simulink model "electricVehicle_closedLoop"  (R2015a)
settings: Solver=ode23t  StartTime=0.0  StopTime=100  RelTol=1e-3  AbsTol=1e-3
PreLoadFcn:
  | car_tire_data
  | load engine_data
undefined symbols (not defined in the file or in its folder): rider_mass, sigbuilder_block, tire_dia, vehicle_mass
libraries: fl_lib x118, nesl_utility x16, sdl_lib x11, simulink x4, elec_lib x1
(part 1 of 2)
settings Model: Creator=sseshadr  LastModifiedBy=chahn
settings SimscapeCC: SimscapeLogType=all  SimscapeLogDataHistory=10000

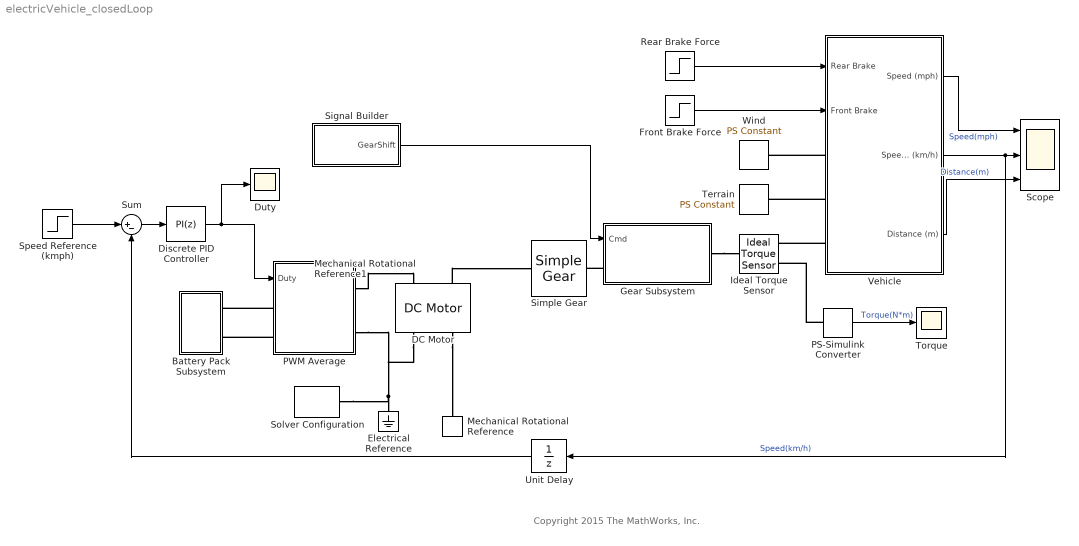
== system electricVehicle_closedLoop ==
  note: Copyright 2015 The MathWorks, Inc.
  Battery Pack Subsystem : Subsystem
  DC Motor : elec_lib/Actuators & Drivers/Rotational Actuators/DC Motor  parameterization=1  Ra=0.0093 Ohm  La=172 uH  emf_or_torque=2  Kv=0.19 V/(rad/s)  Ki=0.19 N*m/A  T_stall=2.4e-4 N*m  w_max=1.91e+4 rpm  w_rated=1.5e+4 rpm  P_rated=0.08 W  V_rated=1.5 V  J=0.001 kg*m^2  lam_param=1  lam=1e-6 N*m/(rad/s)  i_noload=0 A  V_i_noload=1.5 V  speed0=0 rad/s  alpha=0.00393 1/K  Tmeas=25 C  thermal_mass=100 J/K  initial_temperature=25 C
  Discrete PID Controller : simulink/Continuous/PID Controller  Controller=PI  TimeDomain=Discrete-time  SampleTime=0.05  IntegratorMethod=Forward Euler  FilterMethod=Forward Euler  Form=Parallel  UseFilter=on  ControllerParametersSource=internal  P=0.1  I=0.05  D=0  N=100  InitialConditionSource=internal  InitialConditionForIntegrator=0  InitialConditionForFilter=0  ExternalReset=none  LimitOutput=on  UpperSaturationLimit=1  LowerSaturationLimit=0  LinearizeAsGain=off  AntiWindupMode=none  Kb=1  TrackingMode=off  Kt=1  PParamMin=[]  PParamMax=[]  IParamMin=[]  IParamMax=[]  DParamMin=[]  DParamMax=[]  NParamMin=[]  NParamMax=[]  KbParamMin=[]  KbParamMax=[]  KtParamMin=[]  KtParamMax=[]  POutMin=[]  POutMax=[]  IOutMin=[]  IOutMax=[]  DOutMin=[]  DOutMax=[]  NOutMin=[]  NOutMax=[]  KbOutMin=[]  KbOutMax=[]  KtOutMin=[]  KtOutMax=[]  IntegratorOutMin=[]  IntegratorOutMax=[]  FilterOutMin=[]  FilterOutMax=[]  SumOutMin=[]  SumOutMax=[]  SumI1OutMin=[]  SumI1OutMax=[]  SumI2OutMin=[]  SumI2OutMax=[]  SumI3OutMin=[]  SumI3OutMax=[]  SumDOutMin=[]  SumDOutMax=[]  SaturationOutMin=[]  SaturationOutMax=[]  IntegratorContinuousStateAttributes=''  IntegratorStateMustResolveToSignalObject=off  IntegratorRTWStateStorageClass=Auto  FilterContinuousStateAttributes=''  FilterStateMustResolveToSignalObject=off  FilterRTWStateStorageClass=Auto  DifferentiatorICPrevScaledInput=0  DifferentiatorOutMin=[]  DifferentiatorOutMax=[]
  Duty : Scope
      settings: TimeRange=40  LimitDataPoints=on  MaxDataPoints=5000  SaveToWorkspace=off  SaveName=ScopeData4  YMin=0  YMax=1000  SampleTime=-1
  Electrical Reference : fl_lib/Electrical/Electrical Elements/Electrical Reference
  Front Brake Force : Step  Time=75  After=1000  SampleTime=0
      settings: AttributesFormatString=%<After> N at %<Time> s
  Gear Subsystem : Subsystem
  Ideal Torque Sensor : fl_lib/Mechanical/Mechanical Sensors/Ideal Torque Sensor
  Mechanical Rotational Reference : fl_lib/Mechanical/Rotational Elements/Mechanical Rotational Reference
  Mechanical Rotational Reference1 : fl_lib/Mechanical/Rotational Elements/Mechanical Rotational Reference
  PS-Simulink Converter : nesl_utility/PS-Simulink Converter  PhysicalDomain=network_engine_domain  SubClassName=ps_output  LeftPortType=input  RightPortType=output  PseudoPeriodic=off  Frequencies=[]  Unit=N*m  AffineConversion=off
  PWM Average : Subsystem
  Rear Brake Force : Step  Time=50  After=500  SampleTime=0
      settings: AttributesFormatString=%<After> N at %<Time> s
  Scope : Scope  NumInputPorts=3
      settings: TimeRange=auto  MaxDataPoints=5000  SaveToWorkspace=off  YMin=-5~-5~-5  YMax=5~5~5  SampleTime=-1  DataFormat=Array
  Signal Builder : Subsystem  Tag=STV Subsys  LoadFcn=sigbuilder_block('load');  StartFcn=sigbuilder_block('start');  StopFcn=sigbuilder_block('stop');  ClipboardFcn=sigbuilder_block('clipboard');  mask(Sigbuilder block){}
      mask help: Simulink:masks:SigbuilderBlock_MD
      mask init:
      | if ~strcmp(get_param(bdroot(gcbh),'SimulationStatus'),'stopped') tuvar = sigbuilder_block('maskInit'); end
      settings: CopyFcn=sigbuilder_block('copy');  DeleteFcn=sigbuilder_block('delete');  ModelCloseFcn=sigbuilder_block('modelClose');  PreSaveFcn=sigbuilder_block('preSave');  PauseFcn=sigbuilder_block('pause');  ContinueFcn=sigbuilder_block('continue');  NameChangeFcn=sigbuilder_block('namechange');  OpenFcn=sigbuilder_block('open',[306 225.75 549.75 399.75 ]);  CloseFcn=sigbuilder_block('close');
      mask Display: plot(0, 0, 100, 100,[2, 2, 32, 32, 2], [68, 8, 8, 68, 68],[32, 2], [38, 38], [32, 19, 2],[53, 60, 44], [32, 17, 17, 2],[16, 16, 31, 31]);txt = getActiveGroup(gcbh);text(2, 100, txt,'verticalAlignment', 'top');
  Simple Gear : sdl_lib/Gears/Simple Gear  ratio=12  rotation_direction=1  friction_model=1  T_noload=0.1 N*m  T_nom=5 N*m  efficiency_nom=0.8  efficiency=0.8  mu_visc=[ 0 0 ] N*m/(rad/s)  w_thr=0.01 rad/s  temperature_TLU=[ 280 300 320 ] K  load_TLU=[ 1 5 10 ] N*m  efficiency_TLU=[ 0.95 0.9 0.85 ]  efficiency_TLU2=[ 0.85 0.8 0.75; 0.95 0.9 0.85; 0.85 0.8 0.7 ]  thermal_mass=50 J/K  T_init=300 K
  Solver Configuration : nesl_utility/Solver Configuration  PhysicalDomain=network_engine_domain  SubClassName=solver  LeftPortType=input  RightPortType=generic  Accelerate=off  Tones=[]  Harmonics=[]  SimulateNoise=off  Profile=off  UseLocalSampling=off  EnableSwitchedLinearOptims=on  FrequencyDomain=off  UseCCode=off  RelTol=0.001  AbsTol=1e-06  MinStep=1e-09  ToWorkspace=off  RevertToSquareIcSolve=off  NumHomotopyIterations=100  PhasorMode=off  PhasorModeNumHarmonics=1  DoDC=off  ResidualTolerance=1e-09  UseLocalSolver=off  LocalSolverChoice=NE_BACKWARD_EULER_ADVANCER  LocalSolverSampleTime=1e-7  DoFixedCost=off  MaxNonlinIter=3  MaxModeIter=2  LinearAlgebra=Sparse  DelaysMemoryBudget=1024  AutomaticFiltering=on  FilteringTimeConstant=0.001
  Speed Reference (kmph) : Step  Time=30  Before=40  After=5  SampleTime=0
      settings: AttributesFormatString=%<Before> to %<After> at %<Time>s
  Sum : Sum  Inputs=|+-
  Terrain : fl_lib/Physical Signals/Sources/PS Constant  constant=0
  Torque : Scope
      settings: TimeRange=40  LimitDataPoints=on  MaxDataPoints=5000  SaveToWorkspace=off  SaveName=ScopeData2  YMin=0  YMax=1000  SampleTime=-1
  Unit Delay : UnitDelay  SampleTime=0.05
  Vehicle : Subsystem
  Wind : fl_lib/Physical Signals/Sources/PS Constant  constant=0
  wires:
  Rear Brake Force/1 -> Vehicle/1(Rear Brake)
  Vehicle/1(Speed (mph)) -> Scope/1  "Speed(mph)"
  Vehicle/2(Speed (km/h)) -> Unit Delay/1, Scope/2  "Speed(km/h)"
  Vehicle/3(Distance (m)) -> Scope/3  "Distance(m)"
  Front Brake Force/1 -> Vehicle/2(Front Brake)
  PS-Simulink Converter/1 -> Torque/1  "Torque(N*m)"
  Signal Builder/1(GearShift) -> Gear Subsystem/1(Cmd)
  Speed Reference (kmph)/1 -> Sum/1
  Sum/1 -> Discrete PID Controller/1
  Discrete PID Controller/1 -> Duty/1, PWM Average/1(Duty)
  Unit Delay/1 -> Sum/2
  connections:
  Vehicle/LConn1 -- Wind/RConn1
  Vehicle/LConn2 -- Terrain/RConn1
  Vehicle/LConn3 -- Ideal Torque Sensor/RConn1
  PS-Simulink Converter/LConn1 -- Ideal Torque Sensor/RConn2
  Gear Subsystem/RConn1 -- Ideal Torque Sensor/LConn1
  DC Motor/LConn2 -- Simple Gear/LConn1
  Gear Subsystem/LConn1 -- Simple Gear/RConn1
  DC Motor/RConn2 -- Mechanical Rotational Reference/LConn1
  Electrical Reference/LConn1 -- Solver Configuration/RConn1 -- DC Motor/RConn1 -- PWM Average/RConn2
  PWM Average/RConn1 -- DC Motor/LConn1
  PWM Average/LConn1 -- Battery Pack Subsystem/RConn1
  PWM Average/LConn2 -- Battery Pack Subsystem/RConn2

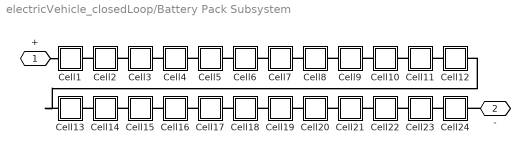
== system electricVehicle_closedLoop/Battery Pack Subsystem ==
  Cell1 : Subsystem
  Cell10 : Subsystem
  Cell11 : Subsystem
  Cell12 : Subsystem
  Cell13 : Subsystem
  Cell14 : Subsystem
  Cell15 : Subsystem
  Cell16 : Subsystem
  Cell17 : Subsystem
  Cell18 : Subsystem
  Cell19 : Subsystem
  Cell2 : Subsystem
  Cell20 : Subsystem
  Cell21 : Subsystem
  Cell22 : Subsystem
  Cell23 : Subsystem
  Cell24 : Subsystem
  Cell3 : Subsystem
  Cell4 : Subsystem
  Cell5 : Subsystem
  Cell6 : Subsystem
  Cell7 : Subsystem
  Cell8 : Subsystem
  Cell9 : Subsystem
  + : PMIOPort  Port=1  Side=Right
  - : PMIOPort  Port=2  Side=Right
  connections:
  +/RConn1 -- Cell1/LConn1
  Cell2/LConn1 -- Cell1/RConn1
  -/RConn1 -- Cell24/RConn1
  Cell3/LConn1 -- Cell2/RConn1
  Cell4/LConn1 -- Cell3/RConn1
  Cell5/LConn1 -- Cell4/RConn1
  Cell6/LConn1 -- Cell5/RConn1
  Cell7/LConn1 -- Cell6/RConn1
  Cell8/LConn1 -- Cell7/RConn1
  Cell9/LConn1 -- Cell8/RConn1
  Cell10/LConn1 -- Cell9/RConn1
  Cell11/LConn1 -- Cell10/RConn1
  Cell12/LConn1 -- Cell11/RConn1
  Cell18/LConn1 -- Cell17/RConn1
  Cell20/LConn1 -- Cell19/RConn1
  Cell15/LConn1 -- Cell14/RConn1
  Cell22/LConn1 -- Cell21/RConn1
  Cell24/LConn1 -- Cell23/RConn1
  Cell23/LConn1 -- Cell22/RConn1
  Cell19/LConn1 -- Cell18/RConn1
  Cell14/LConn1 -- Cell13/RConn1
  Cell21/LConn1 -- Cell20/RConn1
  Cell17/LConn1 -- Cell16/RConn1
  Cell16/LConn1 -- Cell15/RConn1
  Cell13/LConn1 -- Cell12/RConn1

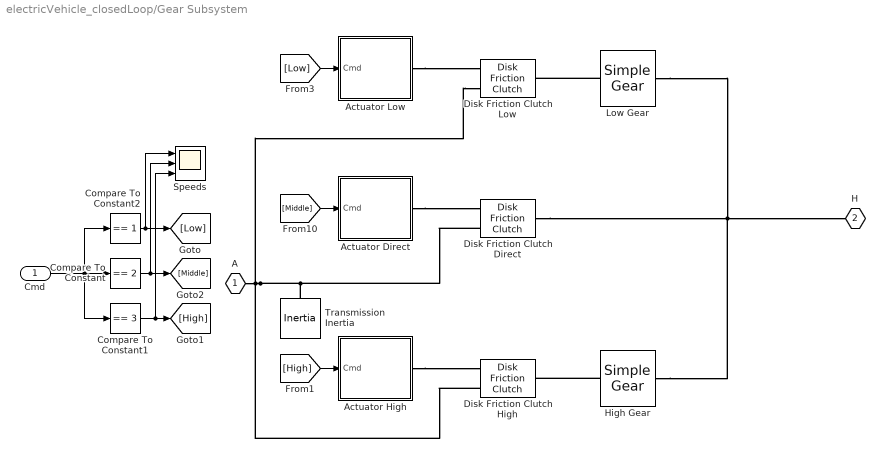
== system electricVehicle_closedLoop/Gear Subsystem ==
  Cmd : Inport
  Actuator Direct : Subsystem
  Actuator High : Subsystem
  Actuator Low : Subsystem
  Compare To Constant : simulink/Logic and Bit Operations/Compare To Constant  relop===  const=2  OutDataTypeStr=boolean
  Compare To Constant1 : simulink/Logic and Bit Operations/Compare To Constant  relop===  const=3  OutDataTypeStr=boolean
  Compare To Constant2 : simulink/Logic and Bit Operations/Compare To Constant  relop===  const=1  OutDataTypeStr=boolean
  Disk Friction Clutch Direct : sdl_lib/Clutches/Disk Friction Clutch  geometry_model=1  r_eff=130 mm  d_o=150 mm  d_i=100 mm  nS=4  piston_area=0.001 m^2  unidirectional=0  friction_model=1  mu_coulomb=0.3  mu_w_vector=[ 0 0.1 0.2 0.3 0.4 0.5 1 2 5 10 100 1000 ] rad/s  mu_coulomb_vector=[ 0.29 0.28 0.26 0.22 0.21 0.2 0.2 0.19 0.19 0.19 0.19 0.19 ]  mu_interp_method=1  mu_extrap_method=1  mu_static=0.35  d_f=1  w_tol=0.001 rad/s  pressure_min=100 Pa  mu_visc=0 N*m/(rad/s)  initial_state_locked=0
  Disk Friction Clutch High : sdl_lib/Clutches/Disk Friction Clutch  geometry_model=1  r_eff=130 mm  d_o=150 mm  d_i=100 mm  nS=4  piston_area=0.001 m^2  unidirectional=0  friction_model=1  mu_coulomb=0.3  mu_w_vector=[ 0 0.1 0.2 0.3 0.4 0.5 1 2 5 10 100 1000 ] rad/s  mu_coulomb_vector=[ 0.29 0.28 0.26 0.22 0.21 0.2 0.2 0.19 0.19 0.19 0.19 0.19 ]  mu_interp_method=1  mu_extrap_method=1  mu_static=0.35  d_f=1  w_tol=0.001 rad/s  pressure_min=100 Pa  mu_visc=0 N*m/(rad/s)  initial_state_locked=0
  Disk Friction Clutch Low : sdl_lib/Clutches/Disk Friction Clutch  geometry_model=1  r_eff=130 mm  d_o=150 mm  d_i=100 mm  nS=4  piston_area=0.001 m^2  unidirectional=0  friction_model=1  mu_coulomb=0.3  mu_w_vector=[ 0 0.1 0.2 0.3 0.4 0.5 1 2 5 10 100 1000 ] rad/s  mu_coulomb_vector=[ 0.29 0.28 0.26 0.22 0.21 0.2 0.2 0.19 0.19 0.19 0.19 0.19 ]  mu_interp_method=1  mu_extrap_method=1  mu_static=0.35  d_f=1  w_tol=0.001 rad/s  pressure_min=100 Pa  mu_visc=0 N*m/(rad/s)  initial_state_locked=0
  High Gear : sdl_lib/Gears/Simple Gear  ratio=0.67  rotation_direction=1  friction_model=1  T_noload=0.1 N*m  T_nom=5 N*m  efficiency_nom=0.8  efficiency=0.8  mu_visc=[ 0 0 ] N*m/(rad/s)  w_thr=0.01 rad/s  temperature_TLU=[ 280 300 320 ] K  load_TLU=[ 1 5 10 ] N*m  efficiency_TLU=[ 0.95 0.9 0.85 ]  efficiency_TLU2=[ 0.85 0.8 0.75; 0.95 0.9 0.85; 0.85 0.8 0.7 ]  thermal_mass=50 J/K  T_init=300 K
  Low Gear : sdl_lib/Gears/Simple Gear  ratio=1.5  rotation_direction=1  friction_model=1  T_noload=0.1 N*m  T_nom=5 N*m  efficiency_nom=0.8  efficiency=0.8  mu_visc=[ 0 0 ] N*m/(rad/s)  w_thr=0.01 rad/s  temperature_TLU=[ 280 300 320 ] K  load_TLU=[ 1 5 10 ] N*m  efficiency_TLU=[ 0.95 0.9 0.85 ]  efficiency_TLU2=[ 0.85 0.8 0.75; 0.95 0.9 0.85; 0.85 0.8 0.7 ]  thermal_mass=50 J/K  T_init=300 K
  Speeds : Scope  NumInputPorts=3
      settings: TimeRange=auto  MaxDataPoints=5000  SaveToWorkspace=off  YMin=-0.2~0~-5  YMax=1.7~2~5  SampleTime=-1
  Transmission Inertia : fl_lib/Mechanical/Rotational Elements/Inertia  inertia=0.0005 kg*m^2  w_specify=off  w_priority=High  w=0 rad/s  t_specify=off  t_priority=High  t=0 N*m
  A : PMIOPort  Port=1  Side=Left
  H : PMIOPort  Port=2  Side=Right
  wires:
  [High] -> Actuator High/1(Cmd)
  [Low] -> Actuator Low/1(Cmd)
  [Middle] -> Actuator Direct/1(Cmd)
  Cmd/1 -> Compare To Constant1/1, Compare To Constant2/1, Compare To Constant/1
  Compare To Constant2/1 -> Speeds/1, [Low]
  Compare To Constant/1 -> Speeds/2, [Middle]
  Compare To Constant1/1 -> Speeds/3, [High]
  connections:
  High Gear/LConn1 -- Disk Friction Clutch High/RConn1
  Actuator High/RConn1 -- Disk Friction Clutch High/LConn1
  Disk Friction Clutch Low/LConn2 -- Disk Friction Clutch High/LConn2 -- Transmission Inertia/LConn1 -- Disk Friction Clutch Direct/LConn2 -- A/RConn1
  Actuator Low/RConn1 -- Disk Friction Clutch Low/LConn1
  Low Gear/LConn1 -- Disk Friction Clutch Low/RConn1
  Actuator Direct/RConn1 -- Disk Friction Clutch Direct/LConn1
  Disk Friction Clutch Direct/RConn1 -- Low Gear/RConn1 -- H/RConn1 -- High Gear/RConn1

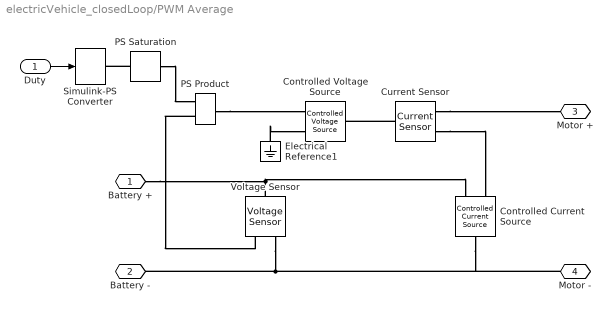
== system electricVehicle_closedLoop/PWM Average ==
  Duty : Inport
  Controlled Current Source : fl_lib/Electrical/Electrical Sources/Controlled Current Source
  Controlled Voltage Source : fl_lib/Electrical/Electrical Sources/Controlled Voltage Source
  Current Sensor : fl_lib/Electrical/Electrical Sensors/Current Sensor
  Electrical Reference1 : fl_lib/Electrical/Electrical Elements/Electrical Reference
  PS Product : fl_lib/Physical Signals/Functions/PS Product
  PS Saturation : fl_lib/Physical Signals/Nonlinear Operators/PS Saturation  upper_limit=1  lower_limit=0
  Simulink-PS Converter : nesl_utility/Simulink-PS Converter  PhysicalDomain=network_engine_domain  SubClassName=ps_input  LeftPortType=input  RightPortType=output  PseudoPeriodic=off  Frequencies=[]  NoiseDistribution=none  NoiseParameters=[]  Unit=1  AffineConversion=off  InputFiltering=off  SimscapeFilterOrder=1  InputFilterTimeConstant=0.001  UdotUserProvided=1
  Voltage Sensor : fl_lib/Electrical/Electrical Sensors/Voltage Sensor
  Battery + : PMIOPort  Port=1  Side=Left
  Battery - : PMIOPort  Port=2  Side=Left
  Motor + : PMIOPort  Port=3  Side=Right
  Motor - : PMIOPort  Port=4  Side=Right
  wires:
  Duty/1 -> Simulink-PS Converter/1
  connections:
  Electrical Reference1/LConn1 -- Controlled Voltage Source/RConn2
  Current Sensor/LConn1 -- Controlled Voltage Source/LConn1
  Voltage Sensor/RConn2 -- Controlled Current Source/LConn1 -- Motor -/RConn1 -- Battery -/RConn1
  Current Sensor/RConn1 -- Controlled Current Source/RConn1
  PS Product/LConn2 -- Voltage Sensor/RConn1
  Voltage Sensor/LConn1 -- Battery +/RConn1 -- Controlled Current Source/RConn2
  PS Product/RConn1 -- Controlled Voltage Source/RConn1
  Current Sensor/RConn2 -- Motor +/RConn1
  PS Saturation/RConn1 -- PS Product/LConn1
  PS Saturation/LConn1 -- Simulink-PS Converter/RConn1

== system electricVehicle_closedLoop/Signal Builder ==
  Demux : Demux  Tag=STV Demux  Outputs=1
  FromWs : FromWorkspace  Tag=STV FromWs  VariableName=tuvar  SampleTime=0
      SigBuilderData=|
      | common.afterFinalStr = 'Extrapolate'
      | common.sampleTime = 0
      | dataSet.timeRange = [0 30]
      | dataSet.name = 'Gear'
      | sbobj.Groups.Name = 'Gear'
      | sbobj.Groups.Signals.Name = 'GearShift'
      | sbobj.Groups.Signals.XData = [0 10 10 20 20 30]
      | sbobj.Groups.Signals.YData = [1 1 2 2 3 3]
      | sbobj.Groups.TimeRange = [0 30]
  GearShift : Outport  Tag=STV Outport
  wires:
  FromWs/1 -> Demux/1
  Demux/1 -> GearShift/1

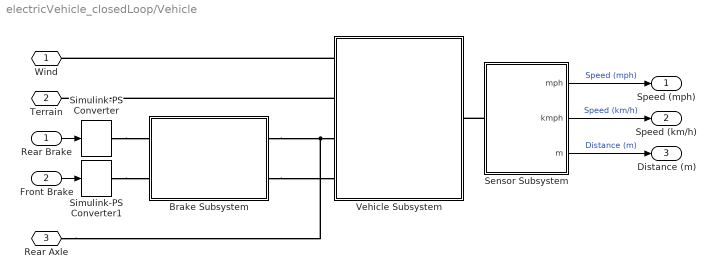
== system electricVehicle_closedLoop/Vehicle ==
  Rear Brake : Inport
  Front Brake : Inport  Port=2
  Brake Subsystem : Subsystem
  Sensor Subsystem : Subsystem
  Simulink-PS Converter : nesl_utility/Simulink-PS Converter  PhysicalDomain=network_engine_domain  SubClassName=ps_input  LeftPortType=input  RightPortType=output  PseudoPeriodic=off  Frequencies=[]  NoiseDistribution=none  NoiseParameters=[]  Unit=1  AffineConversion=off  InputFiltering=on  SimscapeFilterOrder=1  InputFilterTimeConstant=0.001  UdotUserProvided=1
  Simulink-PS Converter1 : nesl_utility/Simulink-PS Converter  PhysicalDomain=network_engine_domain  SubClassName=ps_input  LeftPortType=input  RightPortType=output  PseudoPeriodic=off  Frequencies=[]  NoiseDistribution=none  NoiseParameters=[]  Unit=1  AffineConversion=off  InputFiltering=on  SimscapeFilterOrder=1  InputFilterTimeConstant=0.001  UdotUserProvided=1
  Vehicle Subsystem : Subsystem
  Wind : PMIOPort  Port=1  Side=Left
  Terrain : PMIOPort  Port=2  Side=Left
  Rear Axle : PMIOPort  Port=3  Side=Left
  Speed (mph) : Outport
  Speed (km/h) : Outport  Port=2
  Distance (m) : Outport  Port=3
  wires:
  Sensor Subsystem/1(mph) -> Speed (mph)/1  "Speed (mph)"
  Sensor Subsystem/2(kmph) -> Speed (km/h)/1  "Speed (km/h)"
  Sensor Subsystem/3(m) -> Distance (m)/1  "Distance (m)"
  Rear Brake/1 -> Simulink-PS Converter/1
  Front Brake/1 -> Simulink-PS Converter1/1
  connections:
  Simulink-PS Converter/RConn1 -- Brake Subsystem/LConn1
  Brake Subsystem/RConn1 -- Rear Axle/RConn1 -- Vehicle Subsystem/LConn3
  Brake Subsystem/RConn2 -- Vehicle Subsystem/LConn4
  Simulink-PS Converter1/RConn1 -- Brake Subsystem/LConn2
  Sensor Subsystem/LConn1 -- Vehicle Subsystem/RConn1
  Vehicle Subsystem/LConn1 -- Wind/RConn1
  Vehicle Subsystem/LConn2 -- Terrain/RConn1

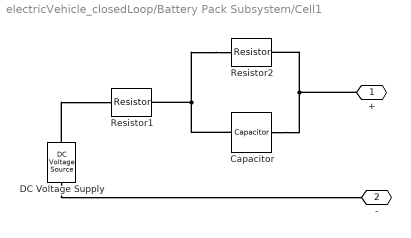
== system electricVehicle_closedLoop/Battery Pack Subsystem/Cell1 ==
  Capacitor : fl_lib/Electrical/Electrical Elements/Capacitor  c=5000 F  r=1e-6 Ohm  g=0 1/Ohm  i_specify=off  i_priority=High  i=0 A  v_specify=off  v_priority=High  v=0 V  vc_specify=on  vc_priority=High  vc=0 V
  DC Voltage Supply : fl_lib/Electrical/Electrical Sources/DC Voltage Source  v0=4.2 V
  Resistor1 : fl_lib/Electrical/Electrical Elements/Resistor  R=0.01 Ohm  i_specify=off  i_priority=High  i=0 A  v_specify=off  v_priority=High  v=0 V
  Resistor2 : fl_lib/Electrical/Electrical Elements/Resistor  R=0.005 Ohm  i_specify=off  i_priority=High  i=0 A  v_specify=off  v_priority=High  v=0 V
  + : PMIOPort  Port=1  Side=Left
  - : PMIOPort  Port=2  Side=Right
  connections:
  Resistor2/LConn1 -- Capacitor/LConn1 -- Resistor1/RConn1
  DC Voltage Supply/RConn1 -- -/RConn1
  Resistor2/RConn1 -- +/RConn1 -- Capacitor/RConn1
  DC Voltage Supply/LConn1 -- Resistor1/LConn1

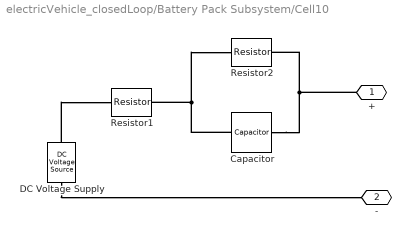
== system electricVehicle_closedLoop/Battery Pack Subsystem/Cell10 ==
  Capacitor : fl_lib/Electrical/Electrical Elements/Capacitor  c=5000 F  r=1e-6 Ohm  g=0 1/Ohm  i_specify=off  i_priority=High  i=0 A  v_specify=off  v_priority=High  v=0 V  vc_specify=on  vc_priority=High  vc=0 V
  DC Voltage Supply : fl_lib/Electrical/Electrical Sources/DC Voltage Source  v0=4.2 V
  Resistor1 : fl_lib/Electrical/Electrical Elements/Resistor  R=0.01 Ohm  i_specify=off  i_priority=High  i=0 A  v_specify=off  v_priority=High  v=0 V
  Resistor2 : fl_lib/Electrical/Electrical Elements/Resistor  R=0.005 Ohm  i_specify=off  i_priority=High  i=0 A  v_specify=off  v_priority=High  v=0 V
  + : PMIOPort  Port=1  Side=Left
  - : PMIOPort  Port=2  Side=Right
  connections:
  DC Voltage Supply/LConn1 -- Resistor1/LConn1
  Capacitor/RConn1 -- +/RConn1 -- Resistor2/RConn1
  DC Voltage Supply/RConn1 -- -/RConn1
  Resistor1/RConn1 -- Capacitor/LConn1 -- Resistor2/LConn1

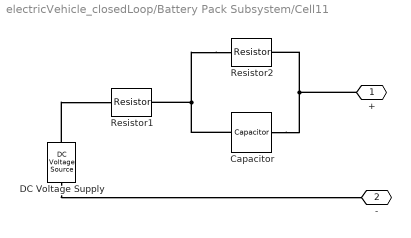
== system electricVehicle_closedLoop/Battery Pack Subsystem/Cell11 ==
  Capacitor : fl_lib/Electrical/Electrical Elements/Capacitor  c=5000 F  r=1e-6 Ohm  g=0 1/Ohm  i_specify=off  i_priority=High  i=0 A  v_specify=off  v_priority=High  v=0 V  vc_specify=on  vc_priority=High  vc=0 V
  DC Voltage Supply : fl_lib/Electrical/Electrical Sources/DC Voltage Source  v0=4.2 V
  Resistor1 : fl_lib/Electrical/Electrical Elements/Resistor  R=0.01 Ohm  i_specify=off  i_priority=High  i=0 A  v_specify=off  v_priority=High  v=0 V
  Resistor2 : fl_lib/Electrical/Electrical Elements/Resistor  R=0.005 Ohm  i_specify=off  i_priority=High  i=0 A  v_specify=off  v_priority=High  v=0 V
  + : PMIOPort  Port=1  Side=Left
  - : PMIOPort  Port=2  Side=Right
  connections:
  Resistor2/LConn1 -- Capacitor/LConn1 -- Resistor1/RConn1
  DC Voltage Supply/RConn1 -- -/RConn1
  Resistor2/RConn1 -- +/RConn1 -- Capacitor/RConn1
  DC Voltage Supply/LConn1 -- Resistor1/LConn1

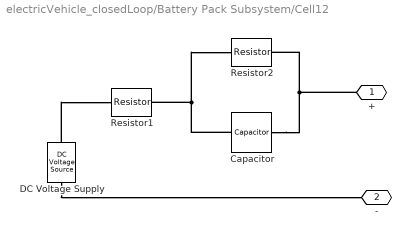
== system electricVehicle_closedLoop/Battery Pack Subsystem/Cell12 ==
  Capacitor : fl_lib/Electrical/Electrical Elements/Capacitor  c=5000 F  r=1e-6 Ohm  g=0 1/Ohm  i_specify=off  i_priority=High  i=0 A  v_specify=off  v_priority=High  v=0 V  vc_specify=on  vc_priority=High  vc=0 V
  DC Voltage Supply : fl_lib/Electrical/Electrical Sources/DC Voltage Source  v0=4.2 V
  Resistor1 : fl_lib/Electrical/Electrical Elements/Resistor  R=0.01 Ohm  i_specify=off  i_priority=High  i=0 A  v_specify=off  v_priority=High  v=0 V
  Resistor2 : fl_lib/Electrical/Electrical Elements/Resistor  R=0.005 Ohm  i_specify=off  i_priority=High  i=0 A  v_specify=off  v_priority=High  v=0 V
  + : PMIOPort  Port=1  Side=Left
  - : PMIOPort  Port=2  Side=Right
  connections:
  DC Voltage Supply/LConn1 -- Resistor1/LConn1
  Capacitor/RConn1 -- +/RConn1 -- Resistor2/RConn1
  DC Voltage Supply/RConn1 -- -/RConn1
  Resistor1/RConn1 -- Capacitor/LConn1 -- Resistor2/LConn1

== system electricVehicle_closedLoop/Battery Pack Subsystem/Cell13 ==
  Capacitor : fl_lib/Electrical/Electrical Elements/Capacitor  c=5000 F  r=1e-6 Ohm  g=0 1/Ohm  i_specify=off  i_priority=High  i=0 A  v_specify=off  v_priority=High  v=0 V  vc_specify=on  vc_priority=High  vc=0 V
  DC Voltage Supply : fl_lib/Electrical/Electrical Sources/DC Voltage Source  v0=4.2 V
  Resistor1 : fl_lib/Electrical/Electrical Elements/Resistor  R=0.01 Ohm  i_specify=off  i_priority=High  i=0 A  v_specify=off  v_priority=High  v=0 V
  Resistor2 : fl_lib/Electrical/Electrical Elements/Resistor  R=0.005 Ohm  i_specify=off  i_priority=High  i=0 A  v_specify=off  v_priority=High  v=0 V
  + : PMIOPort  Port=1  Side=Left
  - : PMIOPort  Port=2  Side=Right
  connections:
  Resistor2/LConn1 -- Capacitor/LConn1 -- Resistor1/RConn1
  DC Voltage Supply/RConn1 -- -/RConn1
  Resistor2/RConn1 -- +/RConn1 -- Capacitor/RConn1
  DC Voltage Supply/LConn1 -- Resistor1/LConn1

== system electricVehicle_closedLoop/Battery Pack Subsystem/Cell14 ==
  Capacitor : fl_lib/Electrical/Electrical Elements/Capacitor  c=5000 F  r=1e-6 Ohm  g=0 1/Ohm  i_specify=off  i_priority=High  i=0 A  v_specify=off  v_priority=High  v=0 V  vc_specify=on  vc_priority=High  vc=0 V
  DC Voltage Supply : fl_lib/Electrical/Electrical Sources/DC Voltage Source  v0=4.2 V
  Resistor1 : fl_lib/Electrical/Electrical Elements/Resistor  R=0.01 Ohm  i_specify=off  i_priority=High  i=0 A  v_specify=off  v_priority=High  v=0 V
  Resistor2 : fl_lib/Electrical/Electrical Elements/Resistor  R=0.005 Ohm  i_specify=off  i_priority=High  i=0 A  v_specify=off  v_priority=High  v=0 V
  + : PMIOPort  Port=1  Side=Left
  - : PMIOPort  Port=2  Side=Right
  connections:
  DC Voltage Supply/LConn1 -- Resistor1/LConn1
  Capacitor/RConn1 -- +/RConn1 -- Resistor2/RConn1
  DC Voltage Supply/RConn1 -- -/RConn1
  Resistor1/RConn1 -- Capacitor/LConn1 -- Resistor2/LConn1

== system electricVehicle_closedLoop/Battery Pack Subsystem/Cell15 ==
  Capacitor : fl_lib/Electrical/Electrical Elements/Capacitor  c=5000 F  r=1e-6 Ohm  g=0 1/Ohm  i_specify=off  i_priority=High  i=0 A  v_specify=off  v_priority=High  v=0 V  vc_specify=on  vc_priority=High  vc=0 V
  DC Voltage Supply : fl_lib/Electrical/Electrical Sources/DC Voltage Source  v0=4.2 V
  Resistor1 : fl_lib/Electrical/Electrical Elements/Resistor  R=0.01 Ohm  i_specify=off  i_priority=High  i=0 A  v_specify=off  v_priority=High  v=0 V
  Resistor2 : fl_lib/Electrical/Electrical Elements/Resistor  R=0.005 Ohm  i_specify=off  i_priority=High  i=0 A  v_specify=off  v_priority=High  v=0 V
  + : PMIOPort  Port=1  Side=Left
  - : PMIOPort  Port=2  Side=Right
  connections:
  Resistor2/LConn1 -- Capacitor/LConn1 -- Resistor1/RConn1
  DC Voltage Supply/RConn1 -- -/RConn1
  Resistor2/RConn1 -- +/RConn1 -- Capacitor/RConn1
  DC Voltage Supply/LConn1 -- Resistor1/LConn1

== system electricVehicle_closedLoop/Battery Pack Subsystem/Cell16 ==
  Capacitor : fl_lib/Electrical/Electrical Elements/Capacitor  c=5000 F  r=1e-6 Ohm  g=0 1/Ohm  i_specify=off  i_priority=High  i=0 A  v_specify=off  v_priority=High  v=0 V  vc_specify=on  vc_priority=High  vc=0 V
  DC Voltage Supply : fl_lib/Electrical/Electrical Sources/DC Voltage Source  v0=4.2 V
  Resistor1 : fl_lib/Electrical/Electrical Elements/Resistor  R=0.01 Ohm  i_specify=off  i_priority=High  i=0 A  v_specify=off  v_priority=High  v=0 V
  Resistor2 : fl_lib/Electrical/Electrical Elements/Resistor  R=0.005 Ohm  i_specify=off  i_priority=High  i=0 A  v_specify=off  v_priority=High  v=0 V
  + : PMIOPort  Port=1  Side=Left
  - : PMIOPort  Port=2  Side=Right
  connections:
  DC Voltage Supply/LConn1 -- Resistor1/LConn1
  Capacitor/RConn1 -- +/RConn1 -- Resistor2/RConn1
  DC Voltage Supply/RConn1 -- -/RConn1
  Resistor1/RConn1 -- Capacitor/LConn1 -- Resistor2/LConn1

== system electricVehicle_closedLoop/Battery Pack Subsystem/Cell17 ==
  Capacitor : fl_lib/Electrical/Electrical Elements/Capacitor  c=5000 F  r=1e-6 Ohm  g=0 1/Ohm  i_specify=off  i_priority=High  i=0 A  v_specify=off  v_priority=High  v=0 V  vc_specify=on  vc_priority=High  vc=0 V
  DC Voltage Supply : fl_lib/Electrical/Electrical Sources/DC Voltage Source  v0=4.2 V
  Resistor1 : fl_lib/Electrical/Electrical Elements/Resistor  R=0.01 Ohm  i_specify=off  i_priority=High  i=0 A  v_specify=off  v_priority=High  v=0 V
  Resistor2 : fl_lib/Electrical/Electrical Elements/Resistor  R=0.005 Ohm  i_specify=off  i_priority=High  i=0 A  v_specify=off  v_priority=High  v=0 V
  + : PMIOPort  Port=1  Side=Left
  - : PMIOPort  Port=2  Side=Right
  connections:
  Resistor2/LConn1 -- Capacitor/LConn1 -- Resistor1/RConn1
  DC Voltage Supply/RConn1 -- -/RConn1
  Resistor2/RConn1 -- +/RConn1 -- Capacitor/RConn1
  DC Voltage Supply/LConn1 -- Resistor1/LConn1

== system electricVehicle_closedLoop/Battery Pack Subsystem/Cell18 ==
  Capacitor : fl_lib/Electrical/Electrical Elements/Capacitor  c=5000 F  r=1e-6 Ohm  g=0 1/Ohm  i_specify=off  i_priority=High  i=0 A  v_specify=off  v_priority=High  v=0 V  vc_specify=on  vc_priority=High  vc=0 V
  DC Voltage Supply : fl_lib/Electrical/Electrical Sources/DC Voltage Source  v0=4.2 V
  Resistor1 : fl_lib/Electrical/Electrical Elements/Resistor  R=0.01 Ohm  i_specify=off  i_priority=High  i=0 A  v_specify=off  v_priority=High  v=0 V
  Resistor2 : fl_lib/Electrical/Electrical Elements/Resistor  R=0.005 Ohm  i_specify=off  i_priority=High  i=0 A  v_specify=off  v_priority=High  v=0 V
  + : PMIOPort  Port=1  Side=Left
  - : PMIOPort  Port=2  Side=Right
  connections:
  DC Voltage Supply/LConn1 -- Resistor1/LConn1
  Capacitor/RConn1 -- +/RConn1 -- Resistor2/RConn1
  DC Voltage Supply/RConn1 -- -/RConn1
  Resistor1/RConn1 -- Capacitor/LConn1 -- Resistor2/LConn1

== system electricVehicle_closedLoop/Battery Pack Subsystem/Cell19 ==
  Capacitor : fl_lib/Electrical/Electrical Elements/Capacitor  c=5000 F  r=1e-6 Ohm  g=0 1/Ohm  i_specify=off  i_priority=High  i=0 A  v_specify=off  v_priority=High  v=0 V  vc_specify=on  vc_priority=High  vc=0 V
  DC Voltage Supply : fl_lib/Electrical/Electrical Sources/DC Voltage Source  v0=4.2 V
  Resistor1 : fl_lib/Electrical/Electrical Elements/Resistor  R=0.01 Ohm  i_specify=off  i_priority=High  i=0 A  v_specify=off  v_priority=High  v=0 V
  Resistor2 : fl_lib/Electrical/Electrical Elements/Resistor  R=0.005 Ohm  i_specify=off  i_priority=High  i=0 A  v_specify=off  v_priority=High  v=0 V
  + : PMIOPort  Port=1  Side=Left
  - : PMIOPort  Port=2  Side=Right
  connections:
  Resistor2/LConn1 -- Capacitor/LConn1 -- Resistor1/RConn1
  DC Voltage Supply/RConn1 -- -/RConn1
  Resistor2/RConn1 -- +/RConn1 -- Capacitor/RConn1
  DC Voltage Supply/LConn1 -- Resistor1/LConn1

== system electricVehicle_closedLoop/Battery Pack Subsystem/Cell2 ==
  Capacitor : fl_lib/Electrical/Electrical Elements/Capacitor  c=5000 F  r=1e-6 Ohm  g=0 1/Ohm  i_specify=off  i_priority=High  i=0 A  v_specify=off  v_priority=High  v=0 V  vc_specify=on  vc_priority=High  vc=0 V
  DC Voltage Supply : fl_lib/Electrical/Electrical Sources/DC Voltage Source  v0=4.2 V
  Resistor1 : fl_lib/Electrical/Electrical Elements/Resistor  R=0.01 Ohm  i_specify=off  i_priority=High  i=0 A  v_specify=off  v_priority=High  v=0 V
  Resistor2 : fl_lib/Electrical/Electrical Elements/Resistor  R=0.005 Ohm  i_specify=off  i_priority=High  i=0 A  v_specify=off  v_priority=High  v=0 V
  + : PMIOPort  Port=1  Side=Left
  - : PMIOPort  Port=2  Side=Right
  connections:
  DC Voltage Supply/LConn1 -- Resistor1/LConn1
  Capacitor/RConn1 -- +/RConn1 -- Resistor2/RConn1
  DC Voltage Supply/RConn1 -- -/RConn1
  Resistor1/RConn1 -- Capacitor/LConn1 -- Resistor2/LConn1

== system electricVehicle_closedLoop/Battery Pack Subsystem/Cell20 ==
  Capacitor : fl_lib/Electrical/Electrical Elements/Capacitor  c=5000 F  r=1e-6 Ohm  g=0 1/Ohm  i_specify=off  i_priority=High  i=0 A  v_specify=off  v_priority=High  v=0 V  vc_specify=on  vc_priority=High  vc=0 V
  DC Voltage Supply : fl_lib/Electrical/Electrical Sources/DC Voltage Source  v0=4.2 V
  Resistor1 : fl_lib/Electrical/Electrical Elements/Resistor  R=0.01 Ohm  i_specify=off  i_priority=High  i=0 A  v_specify=off  v_priority=High  v=0 V
  Resistor2 : fl_lib/Electrical/Electrical Elements/Resistor  R=0.005 Ohm  i_specify=off  i_priority=High  i=0 A  v_specify=off  v_priority=High  v=0 V
  + : PMIOPort  Port=1  Side=Left
  - : PMIOPort  Port=2  Side=Right
  connections:
  DC Voltage Supply/LConn1 -- Resistor1/LConn1
  Capacitor/RConn1 -- +/RConn1 -- Resistor2/RConn1
  DC Voltage Supply/RConn1 -- -/RConn1
  Resistor1/RConn1 -- Capacitor/LConn1 -- Resistor2/LConn1

== system electricVehicle_closedLoop/Battery Pack Subsystem/Cell21 ==
  Capacitor : fl_lib/Electrical/Electrical Elements/Capacitor  c=5000 F  r=1e-6 Ohm  g=0 1/Ohm  i_specify=off  i_priority=High  i=0 A  v_specify=off  v_priority=High  v=0 V  vc_specify=on  vc_priority=High  vc=0 V
  DC Voltage Supply : fl_lib/Electrical/Electrical Sources/DC Voltage Source  v0=4.2 V
  Resistor1 : fl_lib/Electrical/Electrical Elements/Resistor  R=0.01 Ohm  i_specify=off  i_priority=High  i=0 A  v_specify=off  v_priority=High  v=0 V
  Resistor2 : fl_lib/Electrical/Electrical Elements/Resistor  R=0.005 Ohm  i_specify=off  i_priority=High  i=0 A  v_specify=off  v_priority=High  v=0 V
  + : PMIOPort  Port=1  Side=Left
  - : PMIOPort  Port=2  Side=Right
  connections:
  Resistor2/LConn1 -- Capacitor/LConn1 -- Resistor1/RConn1
  DC Voltage Supply/RConn1 -- -/RConn1
  Resistor2/RConn1 -- +/RConn1 -- Capacitor/RConn1
  DC Voltage Supply/LConn1 -- Resistor1/LConn1

== system electricVehicle_closedLoop/Battery Pack Subsystem/Cell22 ==
  Capacitor : fl_lib/Electrical/Electrical Elements/Capacitor  c=5000 F  r=1e-6 Ohm  g=0 1/Ohm  i_specify=off  i_priority=High  i=0 A  v_specify=off  v_priority=High  v=0 V  vc_specify=on  vc_priority=High  vc=0 V
  DC Voltage Supply : fl_lib/Electrical/Electrical Sources/DC Voltage Source  v0=4.2 V
  Resistor1 : fl_lib/Electrical/Electrical Elements/Resistor  R=0.01 Ohm  i_specify=off  i_priority=High  i=0 A  v_specify=off  v_priority=High  v=0 V
  Resistor2 : fl_lib/Electrical/Electrical Elements/Resistor  R=0.005 Ohm  i_specify=off  i_priority=High  i=0 A  v_specify=off  v_priority=High  v=0 V
  + : PMIOPort  Port=1  Side=Left
  - : PMIOPort  Port=2  Side=Right
  connections:
  DC Voltage Supply/LConn1 -- Resistor1/LConn1
  Capacitor/RConn1 -- +/RConn1 -- Resistor2/RConn1
  DC Voltage Supply/RConn1 -- -/RConn1
  Resistor1/RConn1 -- Capacitor/LConn1 -- Resistor2/LConn1

== system electricVehicle_closedLoop/Battery Pack Subsystem/Cell23 ==
  Capacitor : fl_lib/Electrical/Electrical Elements/Capacitor  c=5000 F  r=1e-6 Ohm  g=0 1/Ohm  i_specify=off  i_priority=High  i=0 A  v_specify=off  v_priority=High  v=0 V  vc_specify=on  vc_priority=High  vc=0 V
  DC Voltage Supply : fl_lib/Electrical/Electrical Sources/DC Voltage Source  v0=4.2 V
  Resistor1 : fl_lib/Electrical/Electrical Elements/Resistor  R=0.01 Ohm  i_specify=off  i_priority=High  i=0 A  v_specify=off  v_priority=High  v=0 V
  Resistor2 : fl_lib/Electrical/Electrical Elements/Resistor  R=0.005 Ohm  i_specify=off  i_priority=High  i=0 A  v_specify=off  v_priority=High  v=0 V
  + : PMIOPort  Port=1  Side=Left
  - : PMIOPort  Port=2  Side=Right
  connections:
  Resistor2/LConn1 -- Capacitor/LConn1 -- Resistor1/RConn1
  DC Voltage Supply/RConn1 -- -/RConn1
  Resistor2/RConn1 -- +/RConn1 -- Capacitor/RConn1
  DC Voltage Supply/LConn1 -- Resistor1/LConn1

== system electricVehicle_closedLoop/Battery Pack Subsystem/Cell24 ==
  Capacitor : fl_lib/Electrical/Electrical Elements/Capacitor  c=5000 F  r=1e-6 Ohm  g=0 1/Ohm  i_specify=off  i_priority=High  i=0 A  v_specify=off  v_priority=High  v=0 V  vc_specify=on  vc_priority=High  vc=0 V
  DC Voltage Supply : fl_lib/Electrical/Electrical Sources/DC Voltage Source  v0=4.2 V
  Resistor1 : fl_lib/Electrical/Electrical Elements/Resistor  R=0.01 Ohm  i_specify=off  i_priority=High  i=0 A  v_specify=off  v_priority=High  v=0 V
  Resistor2 : fl_lib/Electrical/Electrical Elements/Resistor  R=0.005 Ohm  i_specify=off  i_priority=High  i=0 A  v_specify=off  v_priority=High  v=0 V
  + : PMIOPort  Port=1  Side=Left
  - : PMIOPort  Port=2  Side=Right
  connections:
  DC Voltage Supply/LConn1 -- Resistor1/LConn1
  Capacitor/RConn1 -- +/RConn1 -- Resistor2/RConn1
  DC Voltage Supply/RConn1 -- -/RConn1
  Resistor1/RConn1 -- Capacitor/LConn1 -- Resistor2/LConn1

== system electricVehicle_closedLoop/Battery Pack Subsystem/Cell3 ==
  Capacitor : fl_lib/Electrical/Electrical Elements/Capacitor  c=5000 F  r=1e-6 Ohm  g=0 1/Ohm  i_specify=off  i_priority=High  i=0 A  v_specify=off  v_priority=High  v=0 V  vc_specify=on  vc_priority=High  vc=0 V
  DC Voltage Supply : fl_lib/Electrical/Electrical Sources/DC Voltage Source  v0=4.2 V
  Resistor1 : fl_lib/Electrical/Electrical Elements/Resistor  R=0.01 Ohm  i_specify=off  i_priority=High  i=0 A  v_specify=off  v_priority=High  v=0 V
  Resistor2 : fl_lib/Electrical/Electrical Elements/Resistor  R=0.005 Ohm  i_specify=off  i_priority=High  i=0 A  v_specify=off  v_priority=High  v=0 V
  + : PMIOPort  Port=1  Side=Left
  - : PMIOPort  Port=2  Side=Right
  connections:
  Resistor2/LConn1 -- Capacitor/LConn1 -- Resistor1/RConn1
  DC Voltage Supply/RConn1 -- -/RConn1
  Resistor2/RConn1 -- +/RConn1 -- Capacitor/RConn1
  DC Voltage Supply/LConn1 -- Resistor1/LConn1

== system electricVehicle_closedLoop/Battery Pack Subsystem/Cell4 ==
  Capacitor : fl_lib/Electrical/Electrical Elements/Capacitor  c=5000 F  r=1e-6 Ohm  g=0 1/Ohm  i_specify=off  i_priority=High  i=0 A  v_specify=off  v_priority=High  v=0 V  vc_specify=on  vc_priority=High  vc=0 V
  DC Voltage Supply : fl_lib/Electrical/Electrical Sources/DC Voltage Source  v0=4.2 V
  Resistor1 : fl_lib/Electrical/Electrical Elements/Resistor  R=0.01 Ohm  i_specify=off  i_priority=High  i=0 A  v_specify=off  v_priority=High  v=0 V
  Resistor2 : fl_lib/Electrical/Electrical Elements/Resistor  R=0.005 Ohm  i_specify=off  i_priority=High  i=0 A  v_specify=off  v_priority=High  v=0 V
  + : PMIOPort  Port=1  Side=Left
  - : PMIOPort  Port=2  Side=Right
  connections:
  DC Voltage Supply/LConn1 -- Resistor1/LConn1
  Capacitor/RConn1 -- +/RConn1 -- Resistor2/RConn1
  DC Voltage Supply/RConn1 -- -/RConn1
  Resistor1/RConn1 -- Capacitor/LConn1 -- Resistor2/LConn1

== system electricVehicle_closedLoop/Battery Pack Subsystem/Cell5 ==
  Capacitor : fl_lib/Electrical/Electrical Elements/Capacitor  c=5000 F  r=1e-6 Ohm  g=0 1/Ohm  i_specify=off  i_priority=High  i=0 A  v_specify=off  v_priority=High  v=0 V  vc_specify=on  vc_priority=High  vc=0 V
  DC Voltage Supply : fl_lib/Electrical/Electrical Sources/DC Voltage Source  v0=4.2 V
  Resistor1 : fl_lib/Electrical/Electrical Elements/Resistor  R=0.01 Ohm  i_specify=off  i_priority=High  i=0 A  v_specify=off  v_priority=High  v=0 V
  Resistor2 : fl_lib/Electrical/Electrical Elements/Resistor  R=0.005 Ohm  i_specify=off  i_priority=High  i=0 A  v_specify=off  v_priority=High  v=0 V
  + : PMIOPort  Port=1  Side=Left
  - : PMIOPort  Port=2  Side=Right
  connections:
  Resistor2/LConn1 -- Capacitor/LConn1 -- Resistor1/RConn1
  DC Voltage Supply/RConn1 -- -/RConn1
  Resistor2/RConn1 -- +/RConn1 -- Capacitor/RConn1
  DC Voltage Supply/LConn1 -- Resistor1/LConn1

== system electricVehicle_closedLoop/Battery Pack Subsystem/Cell6 ==
  Capacitor : fl_lib/Electrical/Electrical Elements/Capacitor  c=5000 F  r=1e-6 Ohm  g=0 1/Ohm  i_specify=off  i_priority=High  i=0 A  v_specify=off  v_priority=High  v=0 V  vc_specify=on  vc_priority=High  vc=0 V
  DC Voltage Supply : fl_lib/Electrical/Electrical Sources/DC Voltage Source  v0=4.2 V
  Resistor1 : fl_lib/Electrical/Electrical Elements/Resistor  R=0.01 Ohm  i_specify=off  i_priority=High  i=0 A  v_specify=off  v_priority=High  v=0 V
  Resistor2 : fl_lib/Electrical/Electrical Elements/Resistor  R=0.005 Ohm  i_specify=off  i_priority=High  i=0 A  v_specify=off  v_priority=High  v=0 V
  + : PMIOPort  Port=1  Side=Left
  - : PMIOPort  Port=2  Side=Right
  connections:
  DC Voltage Supply/LConn1 -- Resistor1/LConn1
  Capacitor/RConn1 -- +/RConn1 -- Resistor2/RConn1
  DC Voltage Supply/RConn1 -- -/RConn1
  Resistor1/RConn1 -- Capacitor/LConn1 -- Resistor2/LConn1

== system electricVehicle_closedLoop/Battery Pack Subsystem/Cell7 ==
  Capacitor : fl_lib/Electrical/Electrical Elements/Capacitor  c=5000 F  r=1e-6 Ohm  g=0 1/Ohm  i_specify=off  i_priority=High  i=0 A  v_specify=off  v_priority=High  v=0 V  vc_specify=on  vc_priority=High  vc=0 V
  DC Voltage Supply : fl_lib/Electrical/Electrical Sources/DC Voltage Source  v0=4.2 V
  Resistor1 : fl_lib/Electrical/Electrical Elements/Resistor  R=0.01 Ohm  i_specify=off  i_priority=High  i=0 A  v_specify=off  v_priority=High  v=0 V
  Resistor2 : fl_lib/Electrical/Electrical Elements/Resistor  R=0.005 Ohm  i_specify=off  i_priority=High  i=0 A  v_specify=off  v_priority=High  v=0 V
  + : PMIOPort  Port=1  Side=Left
  - : PMIOPort  Port=2  Side=Right
  connections:
  Resistor2/LConn1 -- Capacitor/LConn1 -- Resistor1/RConn1
  DC Voltage Supply/RConn1 -- -/RConn1
  Resistor2/RConn1 -- +/RConn1 -- Capacitor/RConn1
  DC Voltage Supply/LConn1 -- Resistor1/LConn1

== system electricVehicle_closedLoop/Battery Pack Subsystem/Cell8 ==
  Capacitor : fl_lib/Electrical/Electrical Elements/Capacitor  c=5000 F  r=1e-6 Ohm  g=0 1/Ohm  i_specify=off  i_priority=High  i=0 A  v_specify=off  v_priority=High  v=0 V  vc_specify=on  vc_priority=High  vc=0 V
  DC Voltage Supply : fl_lib/Electrical/Electrical Sources/DC Voltage Source  v0=4.2 V
  Resistor1 : fl_lib/Electrical/Electrical Elements/Resistor  R=0.01 Ohm  i_specify=off  i_priority=High  i=0 A  v_specify=off  v_priority=High  v=0 V
  Resistor2 : fl_lib/Electrical/Electrical Elements/Resistor  R=0.005 Ohm  i_specify=off  i_priority=High  i=0 A  v_specify=off  v_priority=High  v=0 V
  + : PMIOPort  Port=1  Side=Left
  - : PMIOPort  Port=2  Side=Right
  connections:
  DC Voltage Supply/LConn1 -- Resistor1/LConn1
  Capacitor/RConn1 -- +/RConn1 -- Resistor2/RConn1
  DC Voltage Supply/RConn1 -- -/RConn1
  Resistor1/RConn1 -- Capacitor/LConn1 -- Resistor2/LConn1

== system electricVehicle_closedLoop/Battery Pack Subsystem/Cell9 ==
  Capacitor : fl_lib/Electrical/Electrical Elements/Capacitor  c=5000 F  r=1e-6 Ohm  g=0 1/Ohm  i_specify=off  i_priority=High  i=0 A  v_specify=off  v_priority=High  v=0 V  vc_specify=on  vc_priority=High  vc=0 V
  DC Voltage Supply : fl_lib/Electrical/Electrical Sources/DC Voltage Source  v0=4.2 V
  Resistor1 : fl_lib/Electrical/Electrical Elements/Resistor  R=0.01 Ohm  i_specify=off  i_priority=High  i=0 A  v_specify=off  v_priority=High  v=0 V
  Resistor2 : fl_lib/Electrical/Electrical Elements/Resistor  R=0.005 Ohm  i_specify=off  i_priority=High  i=0 A  v_specify=off  v_priority=High  v=0 V
  + : PMIOPort  Port=1  Side=Left
  - : PMIOPort  Port=2  Side=Right
  connections:
  Resistor2/LConn1 -- Capacitor/LConn1 -- Resistor1/RConn1
  DC Voltage Supply/RConn1 -- -/RConn1
  Resistor2/RConn1 -- +/RConn1 -- Capacitor/RConn1
  DC Voltage Supply/LConn1 -- Resistor1/LConn1

== system electricVehicle_closedLoop/Gear Subsystem/Actuator Direct ==
  Cmd : Inport
  Apply P < Pth : Constant  Value=0
  Apply P > P_th : Constant  Value=1e7
  Simulink-PS Converter : nesl_utility/Simulink-PS Converter  PhysicalDomain=network_engine_domain  SubClassName=ps_input  LeftPortType=input  RightPortType=output  PseudoPeriodic=off  Frequencies=[]  NoiseDistribution=none  NoiseParameters=[]  Unit=1  AffineConversion=off  InputFiltering=off  SimscapeFilterOrder=1  InputFilterTimeConstant=0.001  UdotUserProvided=1
  Switch : Switch  Criteria=u2 > Threshold
  Engage : PMIOPort  Port=1  Side=Right
  wires:
  Apply P > P_th/1 -> Switch/1
  Switch/1 -> Simulink-PS Converter/1
  Apply P < Pth/1 -> Switch/3
  Cmd/1 -> Switch/2
  connections:
  Simulink-PS Converter/RConn1 -- Engage/RConn1

== system electricVehicle_closedLoop/Gear Subsystem/Actuator High ==
  Cmd : Inport
  Apply P < Pth : Constant  Value=0
  Apply P > P_th : Constant  Value=1e7
  Simulink-PS Converter : nesl_utility/Simulink-PS Converter  PhysicalDomain=network_engine_domain  SubClassName=ps_input  LeftPortType=input  RightPortType=output  PseudoPeriodic=off  Frequencies=[]  NoiseDistribution=none  NoiseParameters=[]  Unit=1  AffineConversion=off  InputFiltering=off  SimscapeFilterOrder=1  InputFilterTimeConstant=0.001  UdotUserProvided=1
  Switch : Switch  Criteria=u2 > Threshold
  Engage : PMIOPort  Port=1  Side=Right
  wires:
  Apply P > P_th/1 -> Switch/1
  Switch/1 -> Simulink-PS Converter/1
  Apply P < Pth/1 -> Switch/3
  Cmd/1 -> Switch/2
  connections:
  Simulink-PS Converter/RConn1 -- Engage/RConn1

== system electricVehicle_closedLoop/Gear Subsystem/Actuator Low ==
  Cmd : Inport
  Apply P < Pth : Constant  Value=0
  Apply P > P_th : Constant  Value=1e7
  Simulink-PS Converter : nesl_utility/Simulink-PS Converter  PhysicalDomain=network_engine_domain  SubClassName=ps_input  LeftPortType=input  RightPortType=output  PseudoPeriodic=off  Frequencies=[]  NoiseDistribution=none  NoiseParameters=[]  Unit=1  AffineConversion=off  InputFiltering=off  SimscapeFilterOrder=1  InputFilterTimeConstant=0.001  UdotUserProvided=1
  Switch : Switch  Criteria=u2 > Threshold
  Engage : PMIOPort  Port=1  Side=Right
  wires:
  Cmd/1 -> Switch/2
  Apply P < Pth/1 -> Switch/3
  Switch/1 -> Simulink-PS Converter/1
  Apply P > P_th/1 -> Switch/1
  connections:
  Simulink-PS Converter/RConn1 -- Engage/RConn1

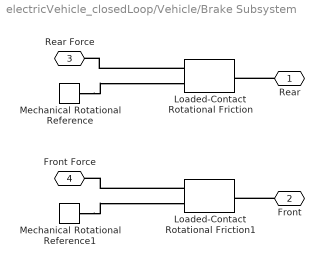
== system electricVehicle_closedLoop/Vehicle/Brake Subsystem ==
  Loaded-Contact Rotational Friction : sdl_lib/Brakes & Detents/Rotational/Loaded-Contact Rotational Friction  geometry_model=1  r_eff=280 mm  d_o=150 mm  d_i=100 mm  friction_model=1  mu_coulomb=0.3  mu_w_vector=[ 0 0.1 0.2 0.3 0.4 0.5 1 2 5 10 100 1000 ] rad/s  mu_coulomb_vector=[ 0.29 0.28 0.26 0.22 0.21 0.2 0.2 0.19 0.19 0.19 0.19 0.19 ]  mu_interp_method=1  mu_extrap_method=1  mu_static=0.35  w_tol=0.001 rad/s  force_min=1 N  mu_visc=0 N*m/(rad/s)  initial_state_locked=0
  Loaded-Contact Rotational Friction1 : sdl_lib/Brakes & Detents/Rotational/Loaded-Contact Rotational Friction  geometry_model=1  r_eff=280 mm  d_o=150 mm  d_i=100 mm  friction_model=1  mu_coulomb=0.3  mu_w_vector=[ 0 0.1 0.2 0.3 0.4 0.5 1 2 5 10 100 1000 ] rad/s  mu_coulomb_vector=[ 0.29 0.28 0.26 0.22 0.21 0.2 0.2 0.19 0.19 0.19 0.19 0.19 ]  mu_interp_method=1  mu_extrap_method=1  mu_static=0.35  w_tol=0.001 rad/s  force_min=1 N  mu_visc=0 N*m/(rad/s)  initial_state_locked=0
  Mechanical Rotational Reference : fl_lib/Mechanical/Rotational Elements/Mechanical Rotational Reference
  Mechanical Rotational Reference1 : fl_lib/Mechanical/Rotational Elements/Mechanical Rotational Reference
  Rear : PMIOPort  Port=1  Side=Right
  Front : PMIOPort  Port=2  Side=Right
  Rear Force : PMIOPort  Port=3  Side=Left
  Front Force : PMIOPort  Port=4  Side=Left
  connections:
  Mechanical Rotational Reference/LConn1 -- Loaded-Contact Rotational Friction/LConn2
  Mechanical Rotational Reference1/LConn1 -- Loaded-Contact Rotational Friction1/LConn2
  Loaded-Contact Rotational Friction/LConn1 -- Rear Force/RConn1
  Loaded-Contact Rotational Friction1/LConn1 -- Front Force/RConn1
  Rear/RConn1 -- Loaded-Contact Rotational Friction/RConn1
  Front/RConn1 -- Loaded-Contact Rotational Friction1/RConn1

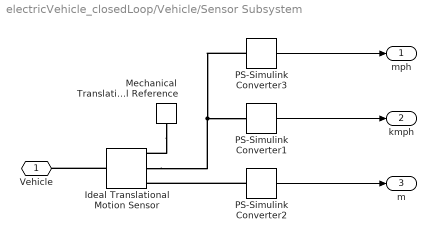
== system electricVehicle_closedLoop/Vehicle/Sensor Subsystem ==
  Ideal Translational Motion Sensor : fl_lib/Mechanical/Mechanical Sensors/Ideal Translational Motion Sensor  offset=0 m
  Mechanical Translational Reference : fl_lib/Mechanical/Translational Elements/Mechanical Translational Reference
  PS-Simulink Converter1 : nesl_utility/PS-Simulink Converter  PhysicalDomain=network_engine_domain  SubClassName=ps_output  LeftPortType=input  RightPortType=output  PseudoPeriodic=off  Frequencies=[]  Unit=km/hr  AffineConversion=off
  PS-Simulink Converter2 : nesl_utility/PS-Simulink Converter  PhysicalDomain=network_engine_domain  SubClassName=ps_output  LeftPortType=input  RightPortType=output  PseudoPeriodic=off  Frequencies=[]  Unit=1  AffineConversion=off
  PS-Simulink Converter3 : nesl_utility/PS-Simulink Converter  PhysicalDomain=network_engine_domain  SubClassName=ps_output  LeftPortType=input  RightPortType=output  PseudoPeriodic=off  Frequencies=[]  Unit=mph  AffineConversion=off
  Vehicle : PMIOPort  Port=1  Side=Left
  mph : Outport
  kmph : Outport  Port=2
  m : Outport  Port=3
  wires:
  PS-Simulink Converter1/1 -> kmph/1
  PS-Simulink Converter2/1 -> m/1
  PS-Simulink Converter3/1 -> mph/1
  connections:
  Mechanical Translational Reference/LConn1 -- Ideal Translational Motion Sensor/RConn1
  PS-Simulink Converter2/LConn1 -- Ideal Translational Motion Sensor/RConn3
  Ideal Translational Motion Sensor/RConn2 -- PS-Simulink Converter3/LConn1 -- PS-Simulink Converter1/LConn1
  Ideal Translational Motion Sensor/LConn1 -- Vehicle/RConn1
